simulink model "wiringmethodpart4"  (R2021b)
settings: Solver=ode15s  StartTime=0.0  StopTime=100  MaxStep=0.002  MinStep=0.000000000000001  RelTol=1e-5
settings Model: Creator=User  LastModifiedBy=User

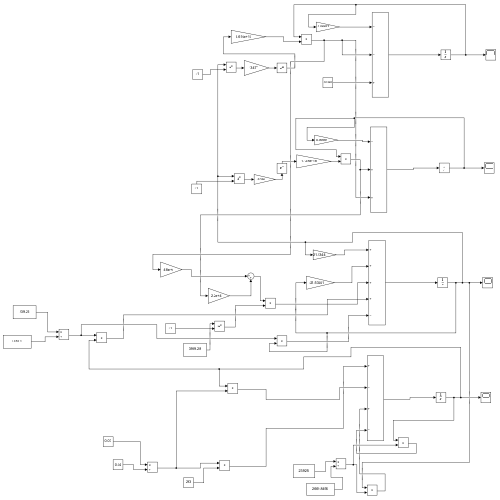
[thumbnail: Simulink's stored preview of the top-level diagram]
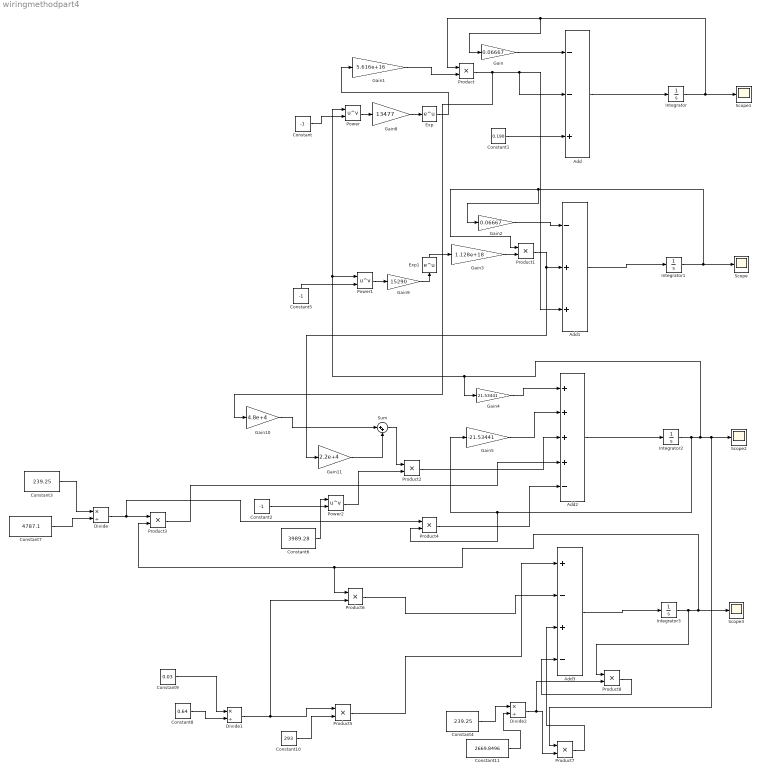
== system wiringmethodpart4 ==
  Add : Sum  Inputs=--+
  Add1 : Sum  Inputs=-++
  Add2 : Sum  Inputs=++++-
  Add3 : Sum  Inputs=+-+-
  Constant : Constant  Value=-1
  Constant1 : Constant  Value=0.190
  Constant10 : Constant  Value=293
  Constant11 : Constant  Value=2669.8496
  Constant2 : Constant  Value=-1
  Constant3 : Constant  Value=239.25
  Constant4 : Constant  Value=239.25
  Constant5 : Constant  Value=-1
  Constant6 : Constant  Value=3989.28
  Constant7 : Constant  Value=4787.1
  Constant8 : Constant  Value=0.64
  Constant9 : Constant  Value=0.03
  Divide : Product  Inputs=*/
  Divide1 : Product  Inputs=*/
  Divide2 : Product  Inputs=*/
  Exp : Math  SaturateOnIntegerOverflow=on
  Exp1 : Math  SaturateOnIntegerOverflow=on
  Gain : Gain  Gain=0.06667
  Gain1 : Gain  Gain=5.616e+16
  Gain10 : Gain  Gain=4.8e+4
  Gain11 : Gain  Gain=2.2e+4
  Gain2 : Gain  Gain=0.06667
  Gain3 : Gain  Gain=1.128e+18
  Gain4 : Gain  Gain=21.53441
  Gain5 : Gain  Gain=-21.53441
  Gain8 : Gain  Gain=13477
  Gain9 : Gain  Gain=15290
  Integrator : Integrator  InitialCondition=0.1649
  Integrator1 : Integrator  InitialCondition=0.9437
  Integrator2 : Integrator  InitialCondition=350.1873
  Integrator3 : Integrator  InitialCondition=330.5469
  Power : Math  Operator=pow  SaturateOnIntegerOverflow=on
  Power1 : Math  Operator=pow  SaturateOnIntegerOverflow=on
  Power2 : Math  Operator=pow  SaturateOnIntegerOverflow=on
  Product{,1..8} (9 alike) : Product
  Scope{,1..3} (4 alike) : Scope
  Sum : Sum  Inputs=|++
  wires:
  Gain/1 -> Add/1
  Constant1/1 -> Add/3
  Add/1 -> Integrator/1
  Integrator/1 -> Scope1/1, Product/1, Gain/1
  Gain1/1 -> Product/2
  Integrator1/1 -> Scope/1, Product1/1, Gain2/1
  Add1/1 -> Integrator1/1
  Product/1 -> Gain10/1, Add1/3, Add/2
  Gain2/1 -> Add1/1
  Gain4/1 -> Add2/1
  Add2/1 -> Integrator2/1
  Gain5/1 -> Add2/2
  Integrator3/1 -> Product8/1, Scope3/1, Product6/1, Product3/2
  Add3/1 -> Integrator3/1
  Constant/1 -> Power/2
  Integrator2/1 -> Product4/2, Gain5/1, Product7/1, Scope2/1, Power/1, Power1/1, Gain4/1
  Power/1 -> Gain8/1
  Gain8/1 -> Exp/1
  Exp/1 -> Gain1/1
  Constant5/1 -> Power1/2
  Power1/1 -> Gain9/1
  Gain9/1 -> Exp1/1
  Exp1/1 -> Gain3/1
  Gain3/1 -> Product1/2
  Product1/1 -> Gain11/1, Add1/2
  Gain10/1 -> Sum/1
  Gain11/1 -> Sum/2
  Constant2/1 -> Power2/2
  Constant6/1 -> Power2/1
  Sum/1 -> Product2/1
  Power2/1 -> Product2/2
  Product2/1 -> Add2/3
  Product3/1 -> Add2/4
  Constant3/1 -> Divide/1
  Constant7/1 -> Divide/2
  Divide/1 -> Product4/1, Product3/1
  Product4/1 -> Add2/5
  Constant8/1 -> Divide1/2
  Constant9/1 -> Divide1/1
  Divide1/1 -> Product6/2, Product5/1
  Constant10/1 -> Product5/2
  Product5/1 -> Add3/1
  Product6/1 -> Add3/2
  Constant4/1 -> Divide2/1
  Constant11/1 -> Divide2/2
  Divide2/1 -> Product8/2, Product7/2
  Product7/1 -> Add3/3
  Product8/1 -> Add3/4
